simulink model "InjCrv_PiI2Set"  (R2016b)
settings: configuration reference "CodeGenConfigSet" (kept outside this file)
values from neighbouring files (symbols this model uses):
  InjCrv_phiPiI2Bas1EOM0_MAP = Calibration.Parameter    [init_InjCrv_PiI2Set.m]    (also in init_InjCrv_PiI2Set_SIL.m = Simulink.Parameter)
  InjCrv_phiPiI2Bas1EOM0_MAPX = Calibration.Parameter    [init_InjCrv_PiI2Set.m]    (also in init_InjCrv_PiI2Set_SIL.m = Simulink.Parameter)
  InjCrv_phiPiI2Bas1EOM0_MAPY = Calibration.Parameter    [init_InjCrv_PiI2Set.m]    (also in init_InjCrv_PiI2Set_SIL.m = Simulink.Parameter)
  InjCrv_qPiI2Bas1EOM0_MAP = Calibration.Parameter    [init_InjCrv_PiI2Set.m]    (also in init_InjCrv_PiI2Set_SIL.m = Simulink.Parameter)
  InjCrv_qPiI2Bas1EOM0_MAPX = Calibration.Parameter    [init_InjCrv_PiI2Set.m]    (also in init_InjCrv_PiI2Set_SIL.m = Simulink.Parameter)
  InjCrv_qPiI2Bas1EOM0_MAPY = Calibration.Parameter    [init_InjCrv_PiI2Set.m]    (also in init_InjCrv_PiI2Set_SIL.m = Simulink.Parameter)
  InjCrv_tiPiI2Bas1EOM0_MAP = Calibration.Parameter    [init_InjCrv_PiI2Set.m]    (also in init_InjCrv_PiI2Set_SIL.m = Simulink.Parameter)
  InjCrv_tiPiI2Bas1EOM0_MAPX = Calibration.Parameter    [init_InjCrv_PiI2Set.m]    (also in init_InjCrv_PiI2Set_SIL.m = Simulink.Parameter)
  InjCrv_tiPiI2Bas1EOM0_MAPY = Calibration.Parameter    [init_InjCrv_PiI2Set.m]    (also in init_InjCrv_PiI2Set_SIL.m = Simulink.Parameter)
settings Model: Creator=Administrator  LastModifiedBy=mayongchao
settings ConfigSetRef: SourceLocation=Base Workspace

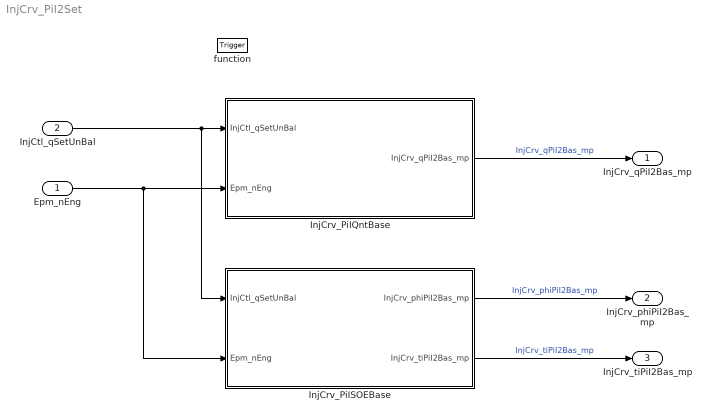
== system InjCrv_PiI2Set ==
  Epm_nEng : Inport  Tag=rpm  Description=Engine speed  OutMin=0  OutMax=6000  OutDataTypeStr=EngSpeed_rpm
  InjCtl_qSetUnBal : Inport  Tag=mg/hub  Description=Current injection quantity  Port=2  OutMin=-319  OutMax=319  OutDataTypeStr=FuelMass_mg_hub
  function : TriggerPort  TriggerType=function-call  VariantControl=Variant
  InjCrv_PiIQntBase : Subsystem  RTWFcnName=InjCrv_PiIQntBase_Co  RTWFileName=InjCrv_PiIQntBase
      settings: RTWSystemCode=Nonreusable function  RTWFcnNameOpts=User specified  RTWFileNameOpts=User specified
  InjCrv_PiISOEBase : Subsystem  RTWFcnName=InjCrv_PiISOEBase_Co  RTWFileName=InjCrv_PiISOEBase
      settings: RTWSystemCode=Nonreusable function  RTWFcnNameOpts=User specified  RTWFileNameOpts=User specified
  InjCrv_qPiI2Bas_mp : Outport  Tag=mg/hub  Description=Basic injection quantity for PiI2  OutMin=-319  OutMax=319  OutDataTypeStr=FuelMass_mg_hub
  InjCrv_phiPiI2Bas_mp : Outport  Tag=CA  Description=Basic PiI2 start of energizing(phi)  Port=2  OutMin=-719  OutMax=719  OutDataTypeStr=Angle_CA
  InjCrv_tiPiI2Bas_mp : Outport  Tag=us  Description=Basic PiI2 start of energizing(ti)  Port=3  OutMin=-13107  OutMax=13106  OutDataTypeStr=InjTime_us
  wires:
  InjCrv_PiIQntBase/1(InjCrv_qPiI2Bas_mp) -> InjCrv_qPiI2Bas_mp/1  "InjCrv_qPiI2Bas_mp"
  InjCrv_PiISOEBase/1(InjCrv_phiPiI2Bas_mp) -> InjCrv_phiPiI2Bas_mp/1  "InjCrv_phiPiI2Bas_mp"
  InjCrv_PiISOEBase/2(InjCrv_tiPiI2Bas_mp) -> InjCrv_tiPiI2Bas_mp/1  "InjCrv_tiPiI2Bas_mp"
  InjCtl_qSetUnBal/1 -> InjCrv_PiISOEBase/1(InjCtl_qSetUnBal), InjCrv_PiIQntBase/1(InjCtl_qSetUnBal)
  Epm_nEng/1 -> InjCrv_PiISOEBase/2(Epm_nEng), InjCrv_PiIQntBase/2(Epm_nEng)

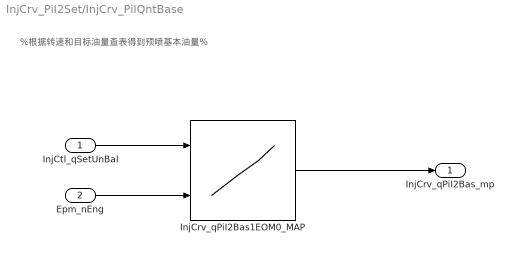
== system InjCrv_PiI2Set/InjCrv_PiIQntBase ==
  note: %根据转速和目标油量查表得到预喷基本油量%
  InjCtl_qSetUnBal : Inport
  Epm_nEng : Inport  Port=2
  InjCrv_qPiI2Bas1EOM0_MAP : Lookup_n-D  BreakpointsForDimension1=InjCrv_qPiI2Bas1EOM0_MAPY  BreakpointsForDimension2=InjCrv_qPiI2Bas1EOM0_MAPX  IndexSearchMethod=Linear search  BeginIndexSearchUsingPreviousIndexResult=on  Table=InjCrv_qPiI2Bas1EOM0_MAP  ExtrapMethod=Clip  UseLastTableValue=on  InternalRulePriority=Speed  OutDataTypeStr=Inherit: Inherit via back propagation  SaturateOnIntegerOverflow=on
  InjCrv_qPiI2Bas_mp : Outport
  wires:
  InjCrv_qPiI2Bas1EOM0_MAP/1 -> InjCrv_qPiI2Bas_mp/1
  InjCtl_qSetUnBal/1 -> InjCrv_qPiI2Bas1EOM0_MAP/1
  Epm_nEng/1 -> InjCrv_qPiI2Bas1EOM0_MAP/2

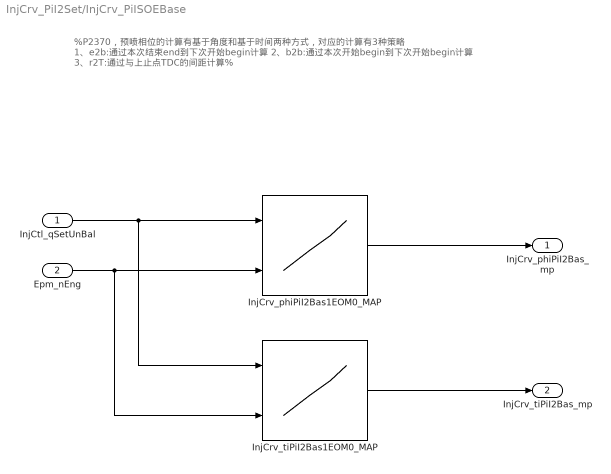
== system InjCrv_PiI2Set/InjCrv_PiISOEBase ==
  note: %P2370，预喷相位的计算有基于角度和基于时间两种方式，对应的计算有3种策略
      | 1、e2b:通过本次结束end到下次开始begin计算
      | 2、b2b:通过本次开始begin到下次开始begin计算
      | 3、r2T:通过与上止点TDC的间距计算%
  InjCtl_qSetUnBal : Inport
  Epm_nEng : Inport  Port=2
  InjCrv_phiPiI2Bas1EOM0_MAP : Lookup_n-D  BreakpointsForDimension1=InjCrv_phiPiI2Bas1EOM0_MAPY  BreakpointsForDimension2=InjCrv_phiPiI2Bas1EOM0_MAPX  IndexSearchMethod=Linear search  BeginIndexSearchUsingPreviousIndexResult=on  Table=InjCrv_phiPiI2Bas1EOM0_MAP  ExtrapMethod=Clip  UseLastTableValue=on  InternalRulePriority=Speed  OutDataTypeStr=Inherit: Inherit via back propagation  SaturateOnIntegerOverflow=on
  InjCrv_tiPiI2Bas1EOM0_MAP : Lookup_n-D  BreakpointsForDimension1=InjCrv_tiPiI2Bas1EOM0_MAPY  BreakpointsForDimension2=InjCrv_tiPiI2Bas1EOM0_MAPX  IndexSearchMethod=Linear search  BeginIndexSearchUsingPreviousIndexResult=on  Table=InjCrv_tiPiI2Bas1EOM0_MAP  ExtrapMethod=Clip  UseLastTableValue=on  InternalRulePriority=Speed  OutDataTypeStr=Inherit: Inherit via back propagation  SaturateOnIntegerOverflow=on
  InjCrv_phiPiI2Bas_mp : Outport
  InjCrv_tiPiI2Bas_mp : Outport  Port=2
  wires:
  InjCrv_tiPiI2Bas1EOM0_MAP/1 -> InjCrv_tiPiI2Bas_mp/1
  InjCrv_phiPiI2Bas1EOM0_MAP/1 -> InjCrv_phiPiI2Bas_mp/1
  InjCtl_qSetUnBal/1 -> InjCrv_tiPiI2Bas1EOM0_MAP/1, InjCrv_phiPiI2Bas1EOM0_MAP/1
  Epm_nEng/1 -> InjCrv_phiPiI2Bas1EOM0_MAP/2, InjCrv_tiPiI2Bas1EOM0_MAP/2
